simulink model "PID_CONTROL_SINGEL"  (Simulink 7.3)
settings: Solver=ode5  StartTime=0.0  StopTime=300  FixedStep=0.01  RelTol=1e-3
libraries: powerlib_extras x1
settings Model: Creator=DANGTHANHBINH  LastModifiedBy=WIN7
settings DebuggingCC: SaveWithParameterizedLinksMsg=none
settings HardwareCC: TargetHWDeviceType=32-bit Generic
settings GRTTargetCC: TargetFcnLib=ansi_tfl_tmw.mat

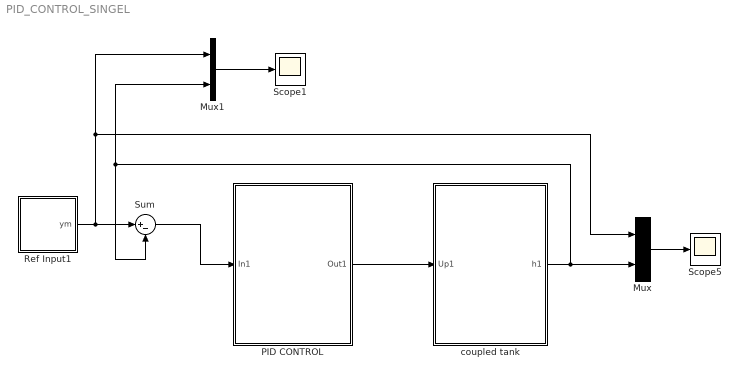
== system PID_CONTROL_SINGEL ==
  Mux : Mux  Inputs=2
  Mux1 : Mux  Inputs=2
  PID CONTROL : Subsystem
  Ref Input1 : Subsystem
  Scope1 : Scope
      settings: SaveName=h1  DataFormat=Array
  Scope5 : Scope
      settings: SaveName=Up  DataFormat=Array
  Sum : Sum  Inputs=|+-  OutDataType=fixdt(1, 16)  OutScaling=2^0
  coupled tank : Subsystem  mask{Kp1=28, a1=0.8, A=85, Cd1=0.6, g=981}
      mask prompts: Kp1 "Kp1   - pump gain1 (cm3/vol.s)"; a1 "a1     - td valve xa1(cm2)"; A "A     - td bon chua (cm2)"; Cd1 "Cd1   - He so xa"; g "g     - Gia toc ttruong"
  wires:
  Mux1/1 -> Scope1/1
  coupled tank/1(h1) -> Mux1/2, Sum/2, Mux/2
  Mux/1 -> Scope5/1
  Ref Input1/1(ym) -> Sum/1, Mux1/1, Mux/1
  PID CONTROL/1(Out1) -> coupled tank/1(Up1)
  Sum/1 -> PID CONTROL/1(In1)

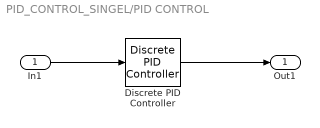
== system PID_CONTROL_SINGEL/PID CONTROL ==
  In1 : Inport  OutDataType=fixdt(1, 16)  OutScaling=2^0
  Discrete PID Controller : powerlib_extras/Discrete  Control Blocks/Discrete PID Controller  DialogController=POWERSYS.PowerSysDialog  SystemSampleTime=-1  Kp=4  Ki=2  Kd=0.2  TcD=1  Par_Limits=[500 -500]  Init=0  Ts=0.01
  Out1 : Outport  OutDataType=fixdt(1, 16)  OutScaling=2^0
  wires:
  In1/1 -> Discrete PID Controller/1
  Discrete PID Controller/1 -> Out1/1

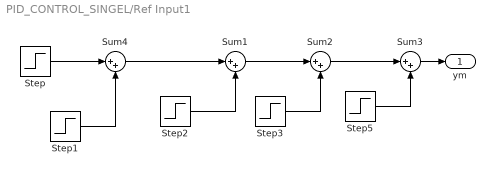
== system PID_CONTROL_SINGEL/Ref Input1 ==
  Step : Step  Time=0  After=35  SampleTime=0
  Step1 : Step  Time=60  After=10  SampleTime=0
  Step2 : Step  Time=120  After=10  SampleTime=0
  Step3 : Step  Time=180  After=-15  SampleTime=0
  Step5 : Step  Time=240  After=10  SampleTime=0
  Sum{1..4} (4 alike) : Sum  Inputs=|++  OutDataType=sfix(16)  OutScaling=2^0  SaturateOnIntegerOverflow=on
  ym : Outport
  wires:
  Step2/1 -> Sum1/2
  Sum1/1 -> Sum2/1
  Step3/1 -> Sum2/2
  Sum2/1 -> Sum3/1
  Step5/1 -> Sum3/2
  Step/1 -> Sum4/1
  Sum4/1 -> Sum1/1
  Sum3/1 -> ym/1
  Step1/1 -> Sum4/2

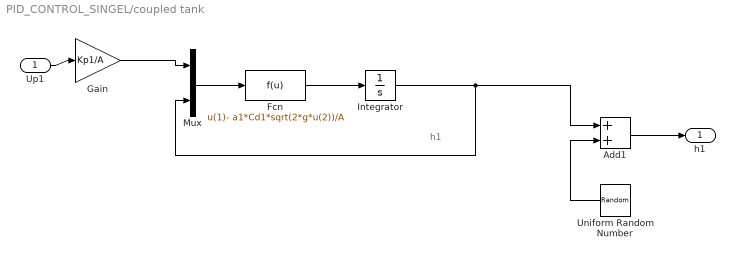
== system PID_CONTROL_SINGEL/coupled tank ==
  note: h1
  Up1 : Inport
  Add1 : Sum  OutDataType=fixdt(1, 16)  OutScaling=2^-10
  Fcn : Fcn  Expr=u(1)- a1*Cd1*sqrt(2*g*u(2))/A
  Gain : Gain  Gain=Kp1/A  ParameterDataType=fixdt(1, 16)  ParameterScaling=2^0  OutDataType=fixdt(1, 16)  OutScaling=2^0
  Integrator : Integrator
  Mux : Mux  Inputs=2
  Uniform Random Number : UniformRandomNumber  Minimum=0  Maximum=0.1  Seed=1234567  SampleTime=0.01
  h1 : Outport
  wires:
  Fcn/1 -> Integrator/1
  Integrator/1 -> Add1/1, Mux/2
  Mux/1 -> Fcn/1
  Up1/1 -> Gain/1
  Gain/1 -> Mux/1
  Add1/1 -> h1/1
  Uniform Random Number/1 -> Add1/2
